simulink library "ssrlib"  (R2021a)
settings: Solver=VariableStepAuto  StartTime=0.0  StopTime=10.0  RelTol=1e-3
settings Model: Creator=sk  LastModifiedBy=sk

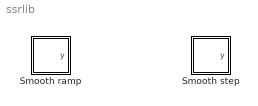
== system ssrlib ==
  Smooth ramp : Subsystem  mask{startTime=1, endTime=2, startValue=0, Slope=1, Smoothness=Jerk/Jolt (3)}
      mask prompts: startTime "Start time"; endTime "End derivative time"; startValue "Initial value"
      mask init:
      | n = double(Smoothness);
      | k = 1:(n-1);
      | A = 1./factorial(n-1+k-k.');
      | y = zeros(n-1,1);
      | y(1) = 1;
      | PolyC = [flip((A\y).'./factorial(n-1+k)) zeros(1,n)];
      mask Display:
      | %plot([.15 .3 .35 .4 .45 .5 .85], [.15 .15 .1597 .1889 0.2375 0.3056 .85])
      | plot([.15 .3  .4  .5 .7 ], [.15 .15 .20 .30 .85])
      | text(.1, .8, num2str(Smoothness))
  Smooth step : Subsystem  mask{startTime=1, endTime=2, startValue=0, endValue=1, Smoothness=Jerk/Jolt (3)}
      mask prompts: startTime "Start time"; endTime "End derivative time"; startValue "Initial value"; endValue "End value"; Smoothness "Function smoothness"
      mask help: Smooth step function
      mask init:
      | n = double(Smoothness);
      | k = 1:n;
      | A = 1./factorial(n+k-k.');
      | y = zeros(n,1);
      | y(1) = 1;
      | PolyC  = [flip((A\y).'./factorial((n-1)+k)) zeros(1,n)];
      mask Display:
      | plot([.15 .3  .4  .5  .6  .85], [.15 .15 .25 .75 .85 .85])
      | text(.1, .8, num2str(Smoothness))

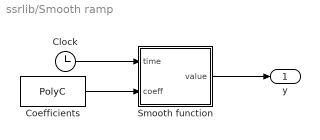
== system ssrlib/Smooth ramp ==
  Clock : Clock
  Coefficients : Constant  Value=PolyC
  Smooth function : MATLAB Function  TreatAsAtomicUnit=on
  y : Outport
  wires:
  Smooth function/1(value) -> y/1
  Clock/1 -> Smooth function/1(time)
  Coefficients/1 -> Smooth function/2(coeff)

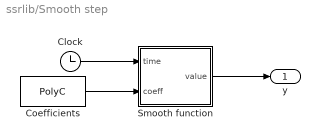
== system ssrlib/Smooth step ==
  Clock : Clock
  Coefficients : Constant  Value=PolyC
  Smooth function : MATLAB Function  TreatAsAtomicUnit=on
  y : Outport
  wires:
  Coefficients/1 -> Smooth function/2(coeff)
  Smooth function/1(value) -> y/1
  Clock/1 -> Smooth function/1(time)

== matlab function ssrlib/Smooth ramp/Smooth function ==
  data: time input double; value output; startTime parameter double size=1; endTime parameter double; startValue parameter double; Slope parameter double; coeff input double
function value = fcn(time, startTime, endTime, startValue, Slope, coeff)
    value = startValue + ...
            Slope .* ...
            arrayfun(@(t, dt) scalarramp(t, dt, coeff), ...
                                time-startTime, endTime-startTime );
end

function y = scalarramp(t, dt, a)
    if t>= dt
        y = t-dt + dt.*polyval(a, 1);
    elseif t <= 0
        y = 0;
    else
        y = dt.*polyval(a, t/dt);
    end
end

== matlab function ssrlib/Smooth step/Smooth function ==
  data: time input double; value output; startTime parameter double size=1; endTime parameter double; startValue parameter double; endValue parameter double; coeff input double
function value = fcn(time, startTime, endTime, startValue, endValue, coeff)
    value = startValue + ...
            endValue .* ...
            arrayfun(@(t, dt) scalarstep(t, dt, coeff), ...
                                time-startTime, endTime-startTime);
end

function y = scalarstep(t, dt, a)
    if t>= dt
        y = 1;
    elseif t <= 0
        y = 0;
    else
        y =  polyval(a, t/dt);
    end
end
